simulink model "FT_property_check"  (R2021b)
settings: Solver=ode45  StartTime=0.0  StopTime=0.2  RelTol=1e-3  EnableMultiTasking=on
undefined symbols (not defined in the file or in its folder): j
settings Model: Creator=my2  LastModifiedBy=82102
settings SolverCC: AlgebraicLoopSolver=TrustRegion
settings DataIOCC: LimitDataPoints=on  SaveFormat=Array  SignalLoggingSaveFormat=ModelDataLogs  ReturnWorkspaceOutputs=off
settings OptimizationCC: LifeSpan=inf
settings DebuggingCC: UnderspecifiedInitializationDetection=Classic  MergeDetectMultiDrivingBlocksExec=none  SolverPrmCheckMsg=warning  FcnCallInpInsideContextMsg=warning  SFUnexpectedBacktrackingDiag=warning  SFNoUnconditionalDefaultTransitionDiag=warning  SFExecutionAtInitializationDiag=none  SFMachineParentedDataDiag=warning  ArithmeticOperatorsInVariantConditions=warning
settings HardwareCC: ProdBitPerPointer=32  ProdBitPerSizeT=32  ProdBitPerPtrDiffT=32  ProdLargestAtomicFloat=None  ProdIntDivRoundTo=Undefined  ProdEndianess=Unspecified  ProdWordSize=32  ProdHWDeviceType=32-bit Generic
settings ModelReferenceCC: PropagateSignalLabelsOutOfModel=off
settings SFSimCC: SimUseLocalCustomCode=off  CustomCodeUndefinedFunction=UseInterfaceOnly
settings RTWCC: RTWUseLocalCustomCode=off
settings CodeAppCC: StateflowObjectComments=on
settings GRTTargetCC: TargetLangStandard=C89/C90 (ANSI)  CombineOutputUpdateFcns=off  GRTInterface=on
settings ConfigComp: CovMetricSettings=dw  CovSaveCumulativeToWorkspaceVar=on  CovSaveSingleToWorkspaceVar=on  CovExternalEMLEnable=off

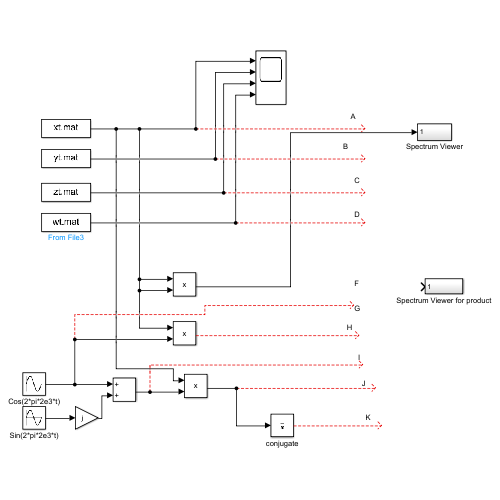
[thumbnail: Simulink's stored preview of the top-level diagram]
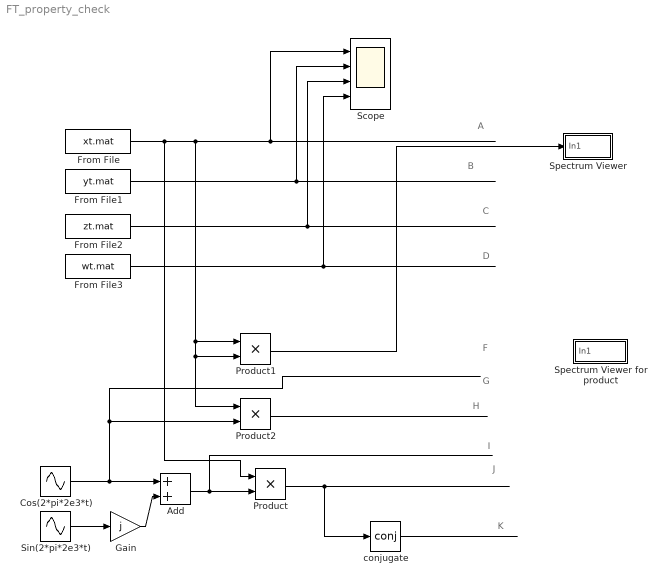
== system FT_property_check ==
  note: A
  note: B
  note: C
  note: D
  note: F
  note: G
  note: H
  note: I
  note: J
  note: K
  Add : Sum
  Cos(2*pi*2e3*t) : Sin  Frequency=2*pi*(2000+5*500)  Phase=pi/2  SampleTime=0
  From File : FromFile  FileName=xt.mat  SampleTime=0
  From File1 : FromFile  FileName=yt.mat  SampleTime=0
  From File2 : FromFile  FileName=zt.mat  SampleTime=0
  From File3 : FromFile  FileName=wt.mat  SampleTime=0
  Gain : Gain  Gain=j
  Product : Product
  Product1 : Product
  Product2 : Product
  Scope : Scope  NumInputPorts=4
  Sin(2*pi*2e3*t) : Sin  Frequency=2*pi*(2000+5*500)  SampleTime=0
  Spectrum Viewer : Subsystem
  Spectrum Viewer for product : Subsystem
  conjugate : Math  Operator=conj  SignedPower=on  SaturateOnIntegerOverflow=on
  wires:
  From File1/1 -> Scope/2
  Sin(2*pi*2e3*t)/1 -> Gain/1
  Cos(2*pi*2e3*t)/1 -> Product2/2, Add/1
  Gain/1 -> Add/2
  Add/1 -> Product/2
  Product/1 -> conjugate/1
  conjugate/1 -> ?
  From File3/1 -> Scope/4
  From File2/1 -> Scope/3
  Product1/1 -> Spectrum Viewer/1(In1)
  From File/1 -> Product/1, Product2/1, Product1/2, Product1/1, Scope/1
  Product2/1 -> ?

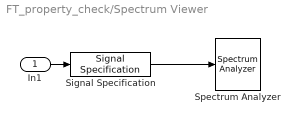
== system FT_property_check/Spectrum Viewer ==
  In1 : Inport
  Signal Specification : SignalSpecification  SampleTime=1/16e3
  Spectrum Analyzer : SpectrumAnalyzer
  wires:
  In1/1 -> Signal Specification/1
  Signal Specification/1 -> Spectrum Analyzer/1

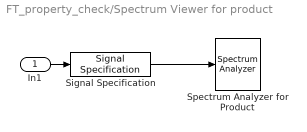
== system FT_property_check/Spectrum Viewer for product ==
  In1 : Inport
  Signal Specification : SignalSpecification  SampleTime=1/16e3
  Spectrum Analyzer for Product : SpectrumAnalyzer
  wires:
  In1/1 -> Signal Specification/1
  Signal Specification/1 -> Spectrum Analyzer for Product/1
